simulink model "untitled"  (R2018b)
settings: Solver=VariableStepAuto  StartTime=0.0  StopTime=10.0  RelTol=1e-3
libraries: fuzblock x1
settings Model: Creator=Jakub  LastModifiedBy=Jakub

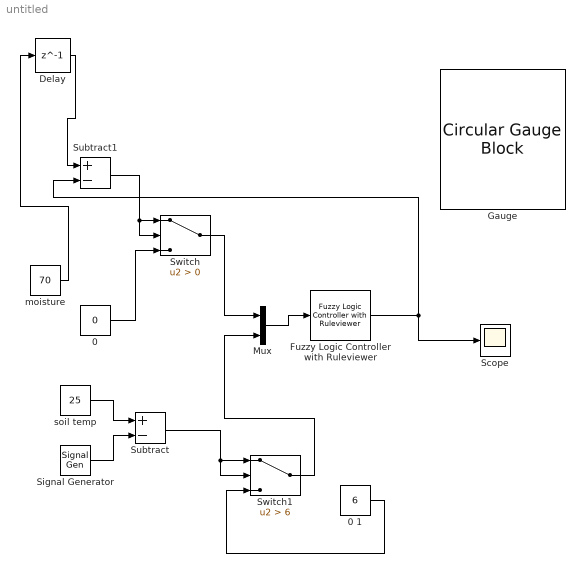
== system untitled ==
  "0 " : Constant  Value=0
  0 1 : Constant  Value=6
  Delay : Delay  DelayLength=1  InitialCondition=0
  Fuzzy Logic Controller with Ruleviewer : fuzblock/Fuzzy Logic  Controller  with Ruleviewer  fismatrix=soil_thresh  Ts=0.1
  Gauge : CircularGaugeBlock  WebBlockId=12  ScaleMin=-300  ScaleMax=1000
  Mux : Mux  Inputs=2
  Scope : Scope
  Signal Generator : SignalGenerator  Amplitude=25  Frequency=0.5  Units=rad/sec
  Subtract : Sum  Inputs=+-
  Subtract1 : Sum  Inputs=+-
  Switch : Switch  Criteria=u2 > Threshold
  Switch1 : Switch  Criteria=u2 > Threshold  Threshold=6
  "moisture " : Constant  Value=70
  "soil temp " : Constant  Value=25
  wires:
  "moisture "/1 -> Delay/1
  "soil temp "/1 -> Subtract/1
  Mux/1 -> Fuzzy Logic Controller with Ruleviewer/1
  Fuzzy Logic Controller with Ruleviewer/1 -> Subtract1/2, Scope/1
  Subtract1/1 -> Switch/2, Switch/1
  Signal Generator/1 -> Subtract/2
  "0 "/1 -> Switch/3
  Switch/1 -> Mux/1
  Delay/1 -> Subtract1/1
  Subtract/1 -> Switch1/2, Switch1/1
  0 1/1 -> Switch1/3
  Switch1/1 -> Mux/2
